simulink model "sample1"  (R2017b)
settings: Solver=VariableStepAuto  StartTime=0.0  StopTime=10.0  RelTol=1e-3
settings Model: Creator=aki  LastModifiedBy=aki

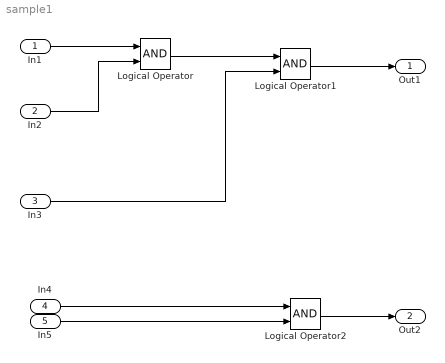
== system sample1 ==
  In1 : Inport
  In2 : Inport  Port=2
  In3 : Inport  Port=3
  In4 : Inport  Port=4
  In5 : Inport  Port=5
  Logical Operator : Logic  AllPortsSameDT=off  OutDataTypeStr=boolean
  Logical Operator1 : Logic  AllPortsSameDT=off  OutDataTypeStr=boolean
  Logical Operator2 : Logic  AllPortsSameDT=off  OutDataTypeStr=boolean
  Out1 : Outport
  Out2 : Outport  Port=2
  wires:
  In1/1 -> Logical Operator/1
  In2/1 -> Logical Operator/2
  Logical Operator/1 -> Logical Operator1/1
  In3/1 -> Logical Operator1/2
  Logical Operator1/1 -> Out1/1
  In4/1 -> Logical Operator2/1
  In5/1 -> Logical Operator2/2
  Logical Operator2/1 -> Out2/1
